simulink model "smc_afr_Controller_autoControls_hw2_q2"  (R2021b)
settings: Solver=VariableStepAuto  StartTime=0.0  StopTime=10.0  RelTol=1e-3
settings Model: Creator=rulij  LastModifiedBy=rulij

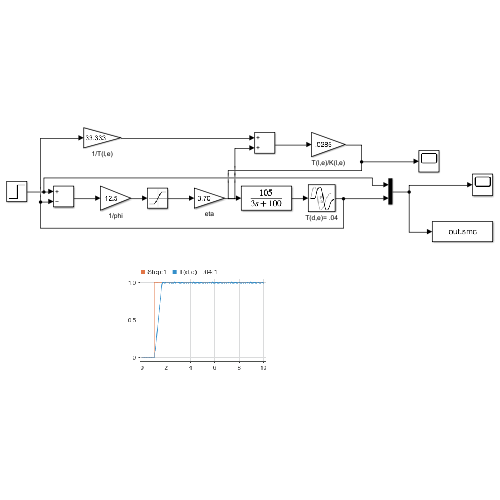
[thumbnail: Simulink's stored preview of the top-level diagram]
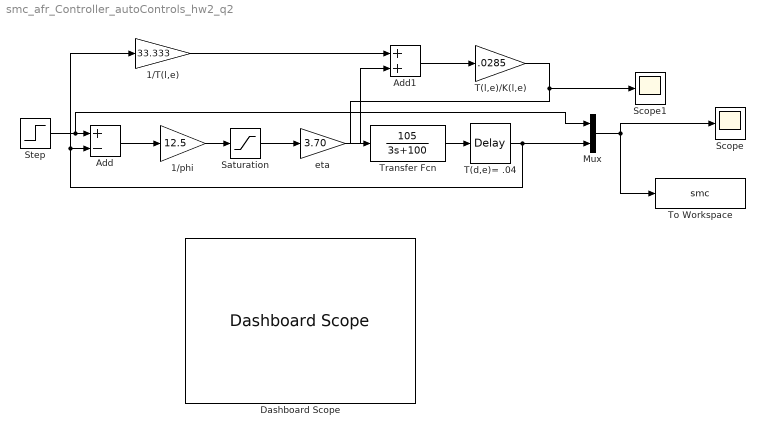
== system smc_afr_Controller_autoControls_hw2_q2 ==
  1/T(l,e) : Gain  Gain=33.333
  1/phi : Gain  Gain=12.5
  Add : Sum  Inputs=+-
  Add1 : Sum
  Dashboard Scope : DashboardScope
  Mux : Mux  Inputs=2
  Saturation : Saturate  UpperLimit=1  LowerLimit=-1
  Scope : Scope
  Scope1 : Scope
  Step : Step  SampleTime=0
  T(d,e)= .04 : TransportDelay  DelayTime=.04
  T(l,e)/K(l,e) : Gain  Gain=.0285
  To Workspace : ToWorkspace  VariableName=smc  SaveFormat=Timeseries  SampleTime=-1
  Transfer Fcn : TransferFcn  Numerator=105  Denominator=[3 100]
  eta : Gain  Gain=3.70
  wires:
  1/phi/1 -> Saturation/1
  Transfer Fcn/1 -> T(d,e)= .04/1
  Mux/1 -> Scope/1, To Workspace/1
  Step/1 -> Mux/1, Add/1
  Add/1 -> 1/phi/1
  Saturation/1 -> eta/1
  eta/1 -> Add1/2
  1/T(l,e)/1 -> Add1/1
  Add1/1 -> T(l,e)/K(l,e)/1
  T(l,e)/K(l,e)/1 -> Scope1/1, Transfer Fcn/1
  T(d,e)= .04/1 -> Add/2, 1/T(l,e)/1, Mux/2
